simulink library "modVehicle000"  (R2018b)
settings: Solver=VariableStepAuto  StartTime=0.0  StopTime=10.0  RelTol=1e-3
undefined symbols (not defined in the file): gndStnMmtArms, lftBdyMmtArms
libraries: turbine_ul x2, vrlib x1, eulAng2RotMat_ul x1, fluidDynamicSurface_cl x1, sixDoFDynamics_ul x1, tethersMoment_cl x1, thrAttachPtKinematics_ul x1
settings Model: Creator=mcobb  LastModifiedBy=jldanie5

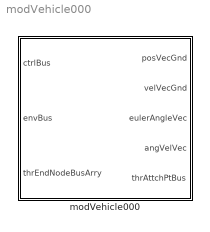
== system modVehicle000 ==
  modVehicle000 : Subsystem  mask{m=1, inertiaMatrix=eye(3), initPos=[0 0 0], initVel=[0 0 0], initEulerAngles=[0 0 0], initAngVel=[0 0 0], rho=1.225, vol=1, grav=9.81, thrAttchStruct=lftBdyMmtArms, CB2CMVec=[1 0 0], turb1Pos=0, turb2Pos=0, turbDiam=0, turbCp=0, turbCd=0, aeroStruct=0}
      mask prompts: m "Mass"; inertiaMatrix "Inertia matrix"; initPos "Initial position vec"; initVel "Initial velocity vec"; initEulerAngles "Initial euler angles"; initAngVel "Initial angular velocity vec"; rho "Fuild Density"; vol "Volume"; grav "Gravity"; thrAttchStruct "Tether attachment struct"; CB2CMVec "CoM 2 CoB Vec"; turb1Pos "Turbine 1 Position Vec"; turb2Pos "Turbine 2 Position Vec"; turbDiam "Diam"; turbCp "Power Coeff"; turbCd "Drag Coeff"; aeroStruct "Fluid dynamic structure"
      mask DialogControl Container9 Prompt: General
      mask DialogControl Container5 Prompt: Inertial Settings
      mask DialogControl ParameterGroupVar Prompt: Environmental
      mask DialogControl Container3 Prompt: Tether attachment positiong vecs in body frame
      mask DialogControl Container4 Prompt: Cent of mass 2 cent of buoy vec
      mask DialogControl Container21 Prompt: Turbines
      mask DialogControl Container22 Prompt: Fluid Dynamics
      mask Display:
      | image('kite.jpg',[100 100 601 528]/4,'on')
      | 
      | port_label('input',1,'ctrlBus')
      | port_label('input',2,'envBus')
      | port_label('input',3,'thrEndNodeBusArry')
      | 
      | port_label('output',1,'posVecGnd')
      | port_label('output',2,'velVecGnd')
      | port_label('output',3,'eulAng')
      | port_label('output',4,'angVelVec')
      | port_label('output',5,'thrAttchPtBus')

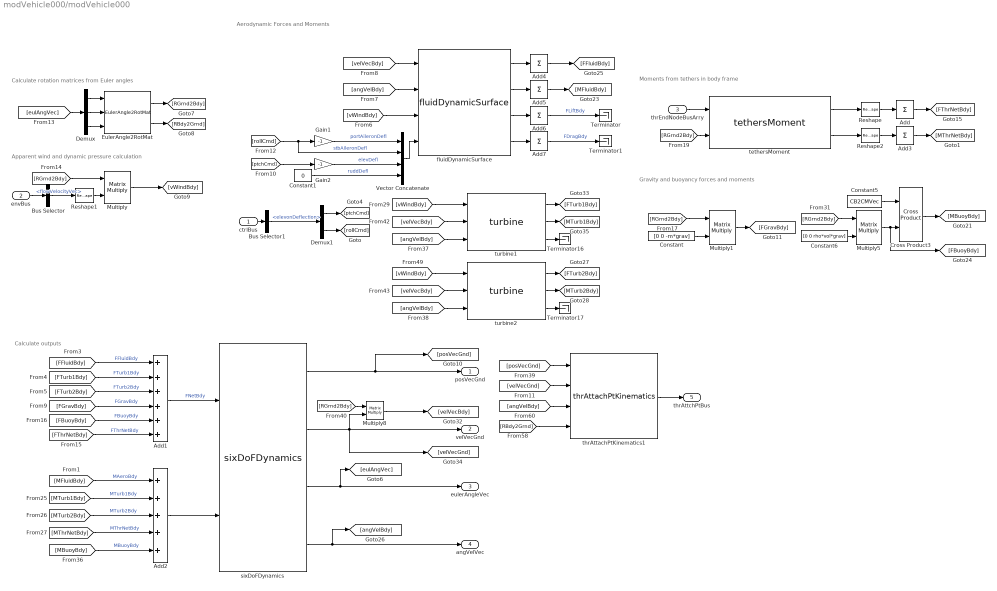
== system modVehicle000/modVehicle000 ==
  note: Calculate outputs
  note: Apparent wind and dynamic pressure calculation
  note: Calculate rotation matrices from Euler angles
  note: Gravity and buoyancy forces and moments
  note: Moments from tethers in body frame
  note: Aerodynamic Forces and Moments
  ctrlBus : Inport  OutDataTypeStr=Bus: ctrlBus
  envBus : Inport  Port=2  OutDataTypeStr=Bus: envBus
  thrEndNodeBusArry : Inport  Port=3
  Add : Sum  Inputs=+  CollapseMode=Specified dimension  CollapseDim=2
  Add1 : Sum  Inputs=++++++
  Add2 : Sum  Inputs=+++++
  Add3 : Sum  Inputs=+  CollapseMode=Specified dimension  CollapseDim=2
  Add{4..7} (4 alike) : Sum  Inputs=1  CollapseMode=Specified dimension  CollapseDim=2
  Bus Selector : BusSelector  OutputSignals=flowVelocityVec
  Bus Selector1 : BusSelector  OutputSignals=elevonDeflection
  Constant : Constant  Value=[0 0 -m*grav]
  Constant1 : Constant  Value=0
  Constant5 : Constant  Value=CB2CMVec
  Constant6 : Constant  Value=[0 0 rho*vol*grav]
  Cross Product3 : vrlib/Utilities/Cross Product
      settings: SourceProductBaseCode=VR
  Demux : Demux  Outputs=3
  Demux1 : Demux  Outputs=2
  EulerAngle2RotMat : eulAng2RotMat_ul/EulerAngle2RotMat  SystemSampleTime=-1
  Gain1 : Gain  Gain=-1
  Gain2 : Gain  Gain=-1
  Multiply{,1,5,8} (4 alike) : Product  Multiplication=Matrix(*)
  Reshape : Reshape  OutputDimensionality=Customize  OutputDimensions=[3 numel(gndStnMmtArms)]
  Reshape1 : Reshape  OutputDimensionality=Column vector (2-D)
  Reshape2 : Reshape  OutputDimensionality=Customize  OutputDimensions=[3 numel(gndStnMmtArms)]
  Terminator{,1,16..17} (4 alike) : Terminator
  Vector Concatenate : Concatenate  NumInputs=4
  fluidDynamicSurface : fluidDynamicSurface_cl/fluidDynamicSurface  aeroStruct=aeroStruct  fluidDensity=rho
  sixDoFDynamics : sixDoFDynamics_ul/sixDoFDynamics  M=m  initPos=initPos  initVel=initVel  J=inertiaMatrix  initEulAngs=initEulerAngles  initAngVel=initAngVel
  tethersMoment : tethersMoment_cl/tethersMoment  arms=thrAttchStruct
  thrAttachPtKinematics1 : thrAttachPtKinematics_ul/thrAttachPtKinematics  atchPts=thrAttchStruct
  turbine1 : turbine_ul/turbine  diam=turbDiam  Cp=turbCp  Cd=turbCd  rho=rho  rTurb=turb1Pos
  turbine2 : turbine_ul/turbine  diam=turbDiam  Cp=turbCp  Cd=turbCd  rho=rho  rTurb=turb2Pos
  posVecGnd : Outport
  velVecGnd : Outport  Port=2
  eulerAngleVec : Outport  Port=3
  angVelVec : Outport  Port=4
  thrAttchPtBus : Outport  Port=5
  wires:
  Bus Selector/1 -> Reshape1/1  "<flowVelocityVec>"
  [eulAngVec] -> Demux/1
  Demux/2 -> EulerAngle2RotMat/2
  Demux/1 -> EulerAngle2RotMat/1
  Demux/3 -> EulerAngle2RotMat/3
  EulerAngle2RotMat/1 -> [RGrnd2Bdy]
  EulerAngle2RotMat/2 -> [RBdy2Grnd]
  [RGrnd2Bdy] -> Multiply/1
  Multiply/1 -> [vWindBdy]
  [RGrnd2Bdy] -> Multiply1/1
  Multiply1/1 -> [FGravBdy]
  thrEndNodeBusArry/1 -> tethersMoment/1
  Constant6/1 -> Multiply5/2
  Multiply5/1 -> Cross Product3/2, [FBuoyBdy]
  [RGrnd2Bdy] -> Multiply5/1
  Cross Product3/1 -> [MBuoyBdy]
  Constant5/1 -> Cross Product3/1
  [MFluidBdy] -> Add2/1  "MAeroBdy"
  [MTurb2Bdy] -> Add2/3  "MTurb2Bdy"
  [MTurb1Bdy] -> Add2/2  "MTurb1Bdy"
  Add2/1 -> sixDoFDynamics/2
  sixDoFDynamics/3 -> [eulAngVec], eulerAngleVec/1
  sixDoFDynamics/4 -> [angVelBdy], angVelVec/1
  turbine1/1 -> [FTurb1Bdy]
  turbine2/1 -> [FTurb2Bdy]
  [FFluidBdy] -> Add1/1  "FFluidBdy"
  [FTurb1Bdy] -> Add1/2  "FTurb1Bdy"
  Constant/1 -> Multiply1/2
  [MBuoyBdy] -> Add2/5  "MBuoyBdy"
  [MThrNetBdy] -> Add2/4  "MThrNetBdy"
  fluidDynamicSurface/2 -> Add5/1
  [FBuoyBdy] -> Add1/5  "FBuoyBdy"
  [FGravBdy] -> Add1/4  "FGravBdy"
  [FTurb2Bdy] -> Add1/3  "FTurb2Bdy"
  [vWindBdy] -> turbine1/1
  turbine1/2 -> [MTurb1Bdy]
  turbine1/3 -> Terminator16/1
  turbine2/2 -> [MTurb2Bdy]
  turbine2/3 -> Terminator17/1
  [angVelBdy] -> turbine1/3
  [vWindBdy] -> turbine2/1
  [angVelBdy] -> turbine2/3
  sixDoFDynamics/1 -> [posVecGnd], posVecGnd/1
  Multiply8/1 -> [velVecBdy]
  sixDoFDynamics/2 -> [velVecGnd], velVecGnd/1, Multiply8/2
  [RGrnd2Bdy] -> Multiply8/1
  [velVecBdy] -> turbine1/2
  [velVecBdy] -> turbine2/2
  [angVelBdy] -> thrAttachPtKinematics1/3
  thrAttachPtKinematics1/1 -> thrAttchPtBus/1
  [posVecGnd] -> thrAttachPtKinematics1/1
  [RBdy2Grnd] -> thrAttachPtKinematics1/4
  [velVecGnd] -> thrAttachPtKinematics1/2
  tethersMoment/1 -> Reshape/1
  Reshape/1 -> Add/1
  Add/1 -> [FThrNetBdy]
  [RGrnd2Bdy] -> tethersMoment/2
  Reshape1/1 -> Multiply/2
  Add3/1 -> [MThrNetBdy]
  Reshape2/1 -> Add3/1
  tethersMoment/2 -> Reshape2/1
  Add1/1 -> sixDoFDynamics/1  "FNetBdy"
  envBus/1 -> Bus Selector/1
  ctrlBus/1 -> Bus Selector1/1
  fluidDynamicSurface/1 -> Add4/1
  fluidDynamicSurface/3 -> Add6/1
  fluidDynamicSurface/4 -> Add7/1
  [vWindBdy] -> fluidDynamicSurface/3
  [angVelBdy] -> fluidDynamicSurface/2
  [velVecBdy] -> fluidDynamicSurface/1
  [FThrNetBdy] -> Add1/6  "FThrNetBdy"
  Vector Concatenate/1 -> fluidDynamicSurface/4
  Bus Selector1/1 -> Demux1/1  "<elevonDeflection>"
  Constant1/1 -> Vector Concatenate/4  "ruddDefl"
  Add4/1 -> [FFluidBdy]
  Add5/1 -> [MFluidBdy]
  Demux1/2 -> [rollCmd]
  Demux1/1 -> [ptchCmd]
  [ptchCmd] -> Gain2/1
  [rollCmd] -> Vector Concatenate/2, Gain1/1  "stbAileronDefl"
  Gain1/1 -> Vector Concatenate/1  "portAileronDefl"
  Gain2/1 -> Vector Concatenate/3  "elevDefl"
  Add6/1 -> Terminator/1  "FLiftBdy"
  Add7/1 -> Terminator1/1  "FDragBdy"
